simulink model "Encoder8_3"  (R2025b)
settings: Solver=VariableStepAuto  StartTime=0.0  StopTime=10.0  RelTol=1e-3
settings Model: Creator=sjpau  LastModifiedBy=Johan

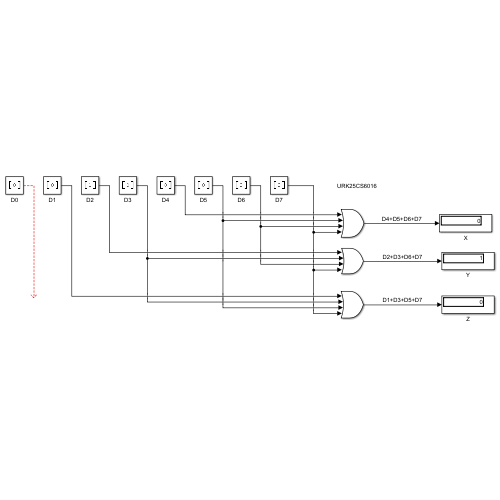
[thumbnail: Simulink's stored preview of the top-level diagram]
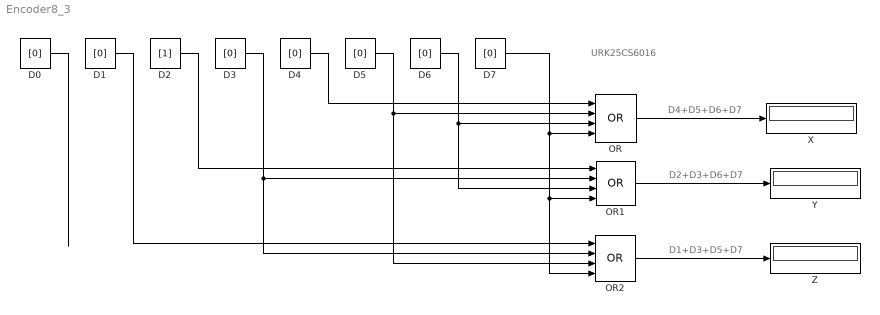
== system Encoder8_3 ==
  note: D4+D5+D6+D7
  note: URK25CS6016
  note: D2+D3+D6+D7
  note: D1+D3+D5+D7
  D{0..1,3..7} (7 alike) : Constant  Value=[0]
  D2 : Constant  Value=[1]
  OR : Logic  Operator=OR  Inputs=4  IconShape=distinctive  AllPortsSameDT=off  OutDataTypeStr=boolean
  OR1 : Logic  Operator=OR  Inputs=4  IconShape=distinctive  AllPortsSameDT=off  OutDataTypeStr=boolean
  OR2 : Logic  Operator=OR  Inputs=4  IconShape=distinctive  AllPortsSameDT=off  OutDataTypeStr=boolean
  X : Display
  Y : Display
  Z : Display
  wires:
  OR2/1 -> Z/1
  OR1/1 -> Y/1
  OR/1 -> X/1
  D7/1 -> OR2/4, OR1/4, OR/4
  D6/1 -> OR1/3, OR/3
  D5/1 -> OR2/3, OR/2
  D4/1 -> OR/1
  D3/1 -> OR2/2, OR1/2
  D2/1 -> OR1/1
  D1/1 -> OR2/1
  D0/1 -> ?
